simulink model "DC2_predistortion"  (R2021b)
settings: Solver=VariableStepAuto  StartTime=0.0  StopTime=30  RelTol=1e-3
model workspace (MATLAB code in the model file):
  | N = 30;
  | sample_time = 0.001;
  | 
  | 
  | A = zeros(N,1);
  | 
  | % x_axis = 0:input_interval:1;
  | 
  | for j=1:1:N+1
  |     A(j) = ((1/N)*j+1)^6 - 1;
  | end
  | 
  | 
  | % boundary_interval = 1/(2*N);
  | %
  | % boundary_vector = [0:boundary_interval:1]';
  | 
  | Gamma = 0.1;
  | K = 0.988;
  | smoothing = 20;
undefined symbols (not defined in the file or in its folder): boundary_vector, magnitude
libraries: commrflib2 x2, dspstat3 x1, commfilt2 x1
settings Model: Creator=paolo  LastModifiedBy=paolo

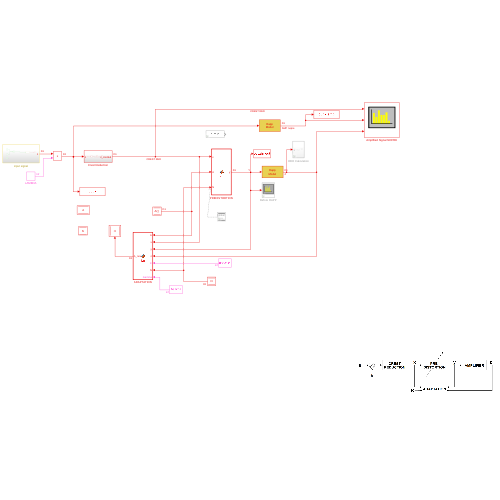
[thumbnail: Simulink's stored preview of the top-level diagram]
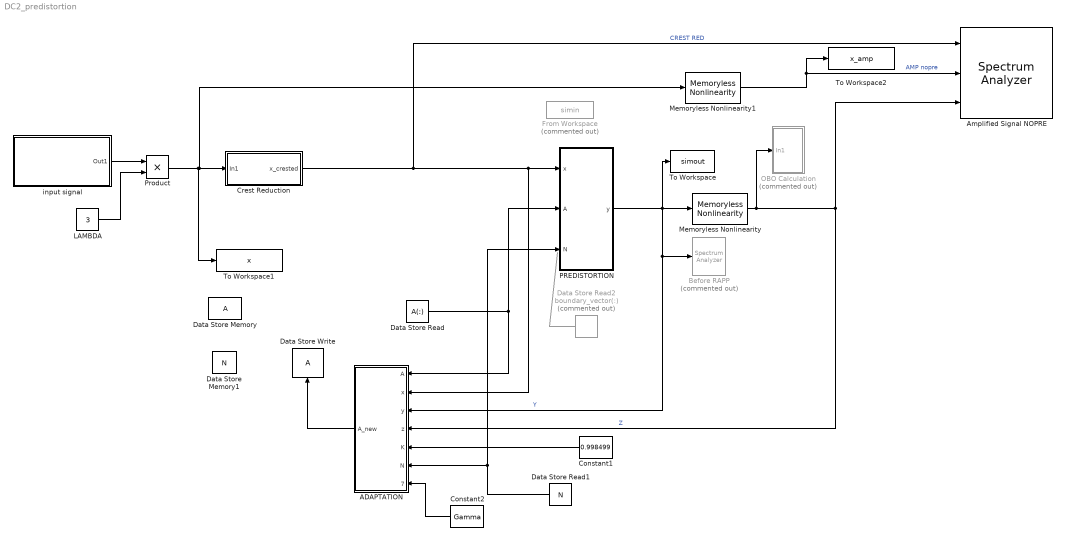
== system DC2_predistortion ==
  ADAPTATION : MATLAB Function  TreatAsAtomicUnit=on
  Amplified Signal NOPRE : SpectrumAnalyzer  NumInputPorts=3
  Before RAPP : SpectrumAnalyzer  Commented=on
  Constant1 : Constant  Value=0.998499
  Constant2 : Constant  Value=Gamma
  Crest Reduction : Subsystem
  Data Store Memory : DataStoreMemory  ReadBeforeWriteMsg=warning  WriteAfterWriteMsg=warning  WriteAfterReadMsg=warning  InitialValue=A  ShowAdditionalParam=off
      settings: SignalType=complex
  Data Store Memory1 : DataStoreMemory  DataStoreName=N  ReadBeforeWriteMsg=warning  WriteAfterWriteMsg=warning  WriteAfterReadMsg=warning  InitialValue=N  ShowAdditionalParam=off  OutDataTypeStr=double
  Data Store Read : DataStoreRead  DataStoreElements=A(:)  IndexOptions=Index vector (dialog)  Indices=1  OutputSizes=1
  Data Store Read1 : DataStoreRead  DataStoreName=N  DataStoreElements=N  IndexOptions=Index vector (dialog)  Indices=1  OutputSizes=1
  Data Store Read2 : DataStoreRead  Commented=on  DataStoreName=boundary_vector  DataStoreElements=boundary_vector(:)  IndexOptions=Index vector (dialog)  Indices=1  OutputSizes=1
  Data Store Write : DataStoreWrite  IndexOptions=Index vector (dialog)  Indices=1  OutputSizes=1
  From Workspace : FromWorkspace  Commented=on  VariableName=simin
  LAMBDA : Constant  Value=3
  Memoryless Nonlinearity : commrflib2/Memoryless Nonlinearity  model_select=Rapp model  linGaindB=0  GindB=0  iip3=30  am2pm=10  LPwrLimAMPM=10  UPwrLimAMPM=inf  amam=[2.1587 1.1517]  ampm=[4.0033 9.1040]  x=[8.1081 1.5413 6.5202 -0.0718]  y=[4.6645 2.0965 10.88 -0.003]  p=smoothing  GoutdB=0  vsat=1
      settings: SourceProductBaseCode=CM
  Memoryless Nonlinearity1 : commrflib2/Memoryless Nonlinearity  model_select=Rapp model  linGaindB=0  GindB=0  iip3=30  am2pm=10  LPwrLimAMPM=10  UPwrLimAMPM=inf  amam=[2.1587 1.1517]  ampm=[4.0033 9.1040]  x=[8.1081 1.5413 6.5202 -0.0718]  y=[4.6645 2.0965 10.88 -0.003]  p=smoothing  GoutdB=0  vsat=1
      settings: SourceProductBaseCode=CM
  OBO Calculation : Subsystem  Commented=on
  PREDISTORTION : MATLAB Function  TreatAsAtomicUnit=on
  Product : Product
  To Workspace : ToWorkspace  VariableName=simout  SaveFormat=Timeseries  SampleTime=-1
  To Workspace1 : ToWorkspace  VariableName=x  SaveFormat=Timeseries  SampleTime=-1
  To Workspace2 : ToWorkspace  VariableName=x_amp  SaveFormat=Timeseries  SampleTime=-1
  input signal : Subsystem
  wires:
  PREDISTORTION/1(y) -> ADAPTATION/3(y), Before RAPP/1, Memoryless Nonlinearity/1, To Workspace/1  "Y"
  Data Store Read1/1 -> ADAPTATION/6(N), PREDISTORTION/3(N)
  Crest Reduction/1(x_crested) -> PREDISTORTION/1(x), ADAPTATION/2(x), Amplified Signal NOPRE/1  "CREST RED"
  Data Store Read/1 -> ADAPTATION/1(A), PREDISTORTION/2(A)
  Product/1 -> Memoryless Nonlinearity1/1, Crest Reduction/1(In1), To Workspace1/1
  Memoryless Nonlinearity/1 -> Amplified Signal NOPRE/3, ADAPTATION/4(z), OBO Calculation/1(In1)  "Z"
  LAMBDA/1 -> Product/2
  input signal/1(Out1) -> Product/1
  Constant2/1 -> ADAPTATION/7(Gamma)
  ADAPTATION/1(A_new) -> Data Store Write/1
  Constant1/1 -> ADAPTATION/5(K)
  Memoryless Nonlinearity1/1 -> To Workspace2/1, Amplified Signal NOPRE/2  "AMP nopre"
  Data Store Read2/1 -> ?

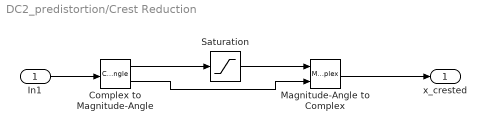
== system DC2_predistortion/Crest Reduction ==
  In1 : Inport
  Complex to Magnitude-Angle : ComplexToMagnitudeAngle
  Magnitude-Angle to Complex : MagnitudeAngleToComplex
  Saturation : Saturate  UpperLimit=1  LowerLimit=-1
  x_crested : Outport
  wires:
  Saturation/1 -> Magnitude-Angle to Complex/1
  Complex to Magnitude-Angle/1 -> Saturation/1
  Complex to Magnitude-Angle/2 -> Magnitude-Angle to Complex/2
  In1/1 -> Complex to Magnitude-Angle/1
  Magnitude-Angle to Complex/1 -> x_crested/1

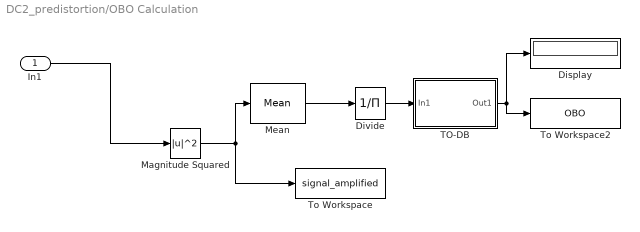
== system DC2_predistortion/OBO Calculation ==
  In1 : Inport
  Display : Display
  Divide : Product  Inputs=/
  Magnitude Squared : Math  Operator=magnitude^2  SaturateOnIntegerOverflow=on
  Mean : dspstat3/Mean  run=on  reset_popup=None  directionMode=Each column  dimension=1  roiEnable=off  roiType=Rectangles  roiPortion=Entire ROI  roiOutput=Individual statistics for each ROI  roiFlag=off  roundingMode=Floor  overflowMode=off  outputDataTypeStr=Inherit: Same as accumulator  outputMin=[]  outputMax=[]  outputLastDataTypeStr=Inherit: Same as accumulator
  TO-DB : Subsystem
  To Workspace : ToWorkspace  VariableName=signal_amplified  SampleTime=-1
      settings: Save2DSignal=2-D array (concatenate along first dimension)
  To Workspace2 : ToWorkspace  VariableName=OBO  SampleTime=-1
      settings: Save2DSignal=2-D array (concatenate along first dimension)
  wires:
  Divide/1 -> TO-DB/1(In1)
  TO-DB/1(Out1) -> Display/1, To Workspace2/1
  In1/1 -> Magnitude Squared/1
  Mean/1 -> Divide/1
  Magnitude Squared/1 -> To Workspace/1, Mean/1

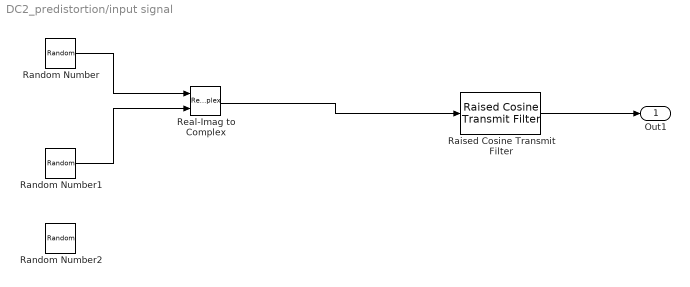
== system DC2_predistortion/input signal ==
  Raised Cosine Transmit Filter : commfilt2/Raised Cosine Transmit Filter  filtType=Square root  R=0.2  filtSpan=10  N=8  filterGain=1  RateOptions=Allow multirate processing  framing=Mute  checkCoeff=off  variableName=rcTxFilt  checkGain=Normalized  sampMode=Mute  saveAsFlag=0  currentFiltSpan=10  D=(10)/2  launchFVT=on  roundingMode=Floor  overflowMode=off  coeffDataTypeStr=Inherit: Same word length as input  coeffMin=[]  coeffMax=[]  coeffLastDataTypeStr=Inherit: Same word length as input  outputDataTypeStr=Inherit: Same as accumulator  outputMin=[]  outputMax=[]  outputLastDataTypeStr=Inherit: Same as accumulator
  Random Number : RandomNumber  Seed=1023  SampleTime=sample_time
  Random Number1 : RandomNumber  Seed=1777  SampleTime=sample_time
  Random Number2 : RandomNumber  Seed=1777  SampleTime=sample_time
  Real-Imag to Complex : RealImagToComplex
  Out1 : Outport
  wires:
  Raised Cosine Transmit Filter/1 -> Out1/1
  Real-Imag to Complex/1 -> Raised Cosine Transmit Filter/1
  Random Number1/1 -> Real-Imag to Complex/2
  Random Number/1 -> Real-Imag to Complex/1

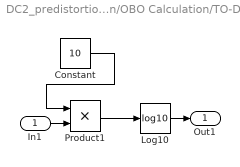
== system DC2_predistortion/OBO Calculation/TO-DB ==
  In1 : Inport
  Constant : Constant  Value=10
  Log10 : Math  Operator=log10  SaturateOnIntegerOverflow=on
  Product1 : Product
  Out1 : Outport
  wires:
  Constant/1 -> Product1/1
  Product1/1 -> Log10/1
  Log10/1 -> Out1/1
  In1/1 -> Product1/2

== matlab function DC2_predistortion/PREDISTORTION ==
  data: x input; y output; A input; N input
function y = fcn(x, A, N)
%#codegen

x_abs = x;
%A_vec = A;

x_abs = abs(x_abs);

n=N+9999;

delta = 1/2*N;

input_interval = 1/N;

%n = N/2;

for i= 1:1:N+1 
    if ( abs(x) > (i-1)*input_interval  ) && ( abs(x) <= (i)*input_interval )
        if (abs(x) - (i-1)*input_interval) < abs(abs(x) - (i)*input_interval)
            n=i;
        else
            n = i+1;
        end
        break
    end
end
    


    a_n = A(n);

    if(n == N+1)
        a_n1 = a_n;
    else 
        a_n1 = A(n+1);
    end
    

    

% denominator = ( x_abs - (n + 1)*delta )*(a_n1 - a_n)
P_x =  ( x_abs - (n + 1)*delta )*(a_n1 - a_n)/( 2*delta) + (a_n1 + a_n)/2;


y= P_x*x;

== matlab function DC2_predistortion/ADAPTATION ==
  data: A input; x input; y input; z input; K input; N input; Gamma input; A_new output
function A_new  = fcn(A, x, y, z, K, N, Gamma)
%#codegen

n = N+100;

% interval_size = max(x_modulus)/2*N;
input_interval = 1/N;



% x
% abs(x)
% A


for i= 1:1:N+1 
    if ( abs(x) > (i-1)*input_interval  ) && ( abs(x) <= (i)*input_interval )
        if (abs(x) - (i-1)*input_interval) < abs(abs(x) - (i)*input_interval)
            n=i;
        else
            n = i+1;
        end
        break
    end
end


A_new1 = A;


A_new1(n) =  A(n) - Gamma*(z - K*x)*(conj(z)/conj(y))*conj(x);


A_new = A_new1;
